simulink model "vexv5_Monitor_Tune_Dashboard"  (R2019a)
settings: Solver=ode3  StartTime=0.0  StopTime=inf  RelTol=1e-3  EnableMultiTasking=on
libraries: vexv5lib x3, vexcommonlib x1
settings Model: SimulationMode=external  ExtModeTrigDuration=25  Creator=The MathWorks, Inc.  LastModifiedBy=josea
settings DataIOCC: LimitDataPoints=on  SaveFormat=Array  ReturnWorkspaceOutputs=off
settings OptimizationCC: ExpressionDepthLimit=2147483647  LifeSpan=Inf  MaxStackSize=64
settings DebuggingCC: UnderspecifiedInitializationDetection=Classic  MergeDetectMultiDrivingBlocksExec=none  InheritedTsInSrcMsg=none  FcnCallInpInsideContextMsg=warning  UnconnectedInputMsg=none  UnconnectedOutputMsg=none  AllowSymbolicDim=off  StateNameClashWarn=warning  PregeneratedLibrarySubsystemCodeDiagnostic=none  SFUnexpectedBacktrackingDiag=warning  SFNoUnconditionalDefaultTransitionDiag=warning  SFExecutionAtInitializationDiag=none  ArithmeticOperatorsInVariantConditions=warning
settings HardwareCC: ProdBitPerPointer=32  ProdBitPerSizeT=32  ProdBitPerPtrDiffT=32  ProdLargestAtomicInteger=Long  ProdLargestAtomicFloat=Double  ProdWordSize=32  ProdHWDeviceType=ARM Compatible->ARM Cortex  UseEmbeddedCoderFeatures=off
settings ModelReferenceCC: PropagateSignalLabelsOutOfModel=off
settings SFSimCC: SimUseLocalCustomCode=off
settings RTWCC: SystemTargetFile=ert.tlc  HardwareBoard=VEX V5 Robot Brain  TLCOptions=-aInlineSetEventsForThisBaseRateFcn=TLC_FALSE -aSuppressMultiTaskScheduler=TLC_FALSE -aRateBasedStepFcn=0  TemplateMakefile=ert_default_tmf  RTWUseLocalCustomCode=off  Toolchain=GNU Tools for ARM Embedded Processors
settings CodeAppCC: StateflowObjectComments=on
settings ERTTargetCC: CodeReplacementLibrary=GCC ARM Cortex-M3  MultiwordLength=2048  ERTCustomFileBanners=off  SupportContinuousTime=on  SupportNonInlinedSFcns=on  RemoveResetFunc=off  ModelStepFunctionPrototypeControlCompliant=off  ConvertIfToSwitch=off  SuppressUnreachableDefaultCases=off
settings ConfigComp: CovMetricSettings=dw  CovHtmlReporting=on  CovSaveCumulativeToWorkspaceVar=on  CovSaveSingleToWorkspaceVar=on  CovExternalEMLEnable=off  CovSFcnEnable=off

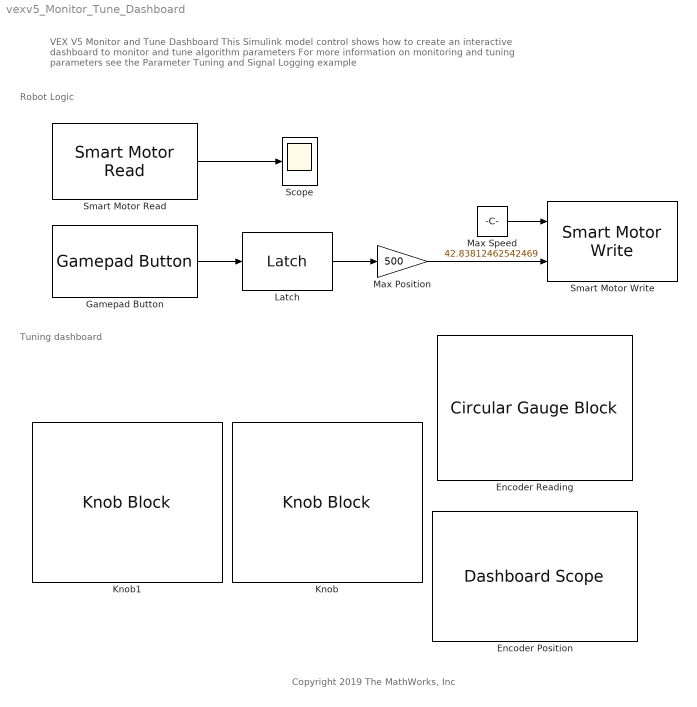
== system vexv5_Monitor_Tune_Dashboard ==
  note: Tuning dashboard
  note: Robot Logic
  note: VEX V5 Monitor and Tune Dashboard
      | This Simulink model control shows how to create an interactive dashboard to monitor and tune algorithm parameters
      | For more information on monitoring and tuning parameters see the Parameter Tuning and Signal Logging example
  note: Copyright 2019 The MathWorks, Inc
  Encoder Position : DashboardScope  Ymin=-100  Ymax=800  LegendPosition=Hide  ScaleAtStop=off
  Encoder Reading : CircularGaugeBlock  LabelPosition=Hide  ScaleMax=600  TickInterval=60
  Gamepad Button : vexv5lib/Gamepad/Gamepad Button  joystickType=Master  chan=X  SampleTime=0.02
      settings: SourceProductName=Simulink Coder Support Package for VEX EDR V5 Robot Brain  SourceProductBaseCode=VEXV5
  Knob : KnobBlock  ScaleMax=50  TickInterval=5
  Knob1 : KnobBlock  ScaleMax=600  TickInterval=50
  Latch : vexcommonlib/Latch  output0=off  BlockPlatform=vexarmcortex
      settings: SourceProductName=Simulink Coder Support Package for ARM Cortex-based VEX Microcontroller  SourceProductBaseCode=EC_VEX_MICRO
  Max Position : Gain  Gain=500
  Max Speed : Constant  Value=42.83812462542469
  Scope : Scope
  Smart Motor Read : vexv5lib/Sensors/Smart Motor Read  motorPort=8  EncoderUnit=Counts  resetOption=No reset  additionalOutput=off  SampleTime=0.05
      settings: SourceProductName=Simulink Coder Support Package for VEX EDR V5 Robot Brain  SourceProductBaseCode=VEXV5
  Smart Motor Write : vexv5lib/Actuators/Smart Motor Write  motorPort=8  scaleFactor=18:1  MotorBrakeMode=Hold  OperationMode=Position Control
      settings: SourceProductName=Simulink Coder Support Package for VEX EDR V5 Robot Brain  SourceProductBaseCode=VEXV5
  wires:
  Gamepad Button/1 -> Latch/1
  Latch/1 -> Max Position/1
  Max Position/1 -> Smart Motor Write/2
  Max Speed/1 -> Smart Motor Write/1
  Smart Motor Read/1 -> Scope/1
